simulink model "Copy_2_of_canceshi"  (Simulink 8.8)
settings: Solver=ode4  StartTime=0.0  StopTime=inf  FixedStep=0.1  RelTol=1e-3  EnableMultiTasking=on
undefined symbols (not defined in the file or in its folder): bit, Standard
libraries: slrtlib x21, slrtsoftinglib x11
CloseFcn:
  | rtwprivate ssgencode ModelCloseRequest canceshi
settings Model: xpc_rtwmakecfg_data=_xpccanac2pci_  Creator=Administrator  LastModifiedBy=15751  SimulationMode=external
settings SolverCC: EnableConcurrentExecution=on
settings OptimizationCC: BlockReduction=off  OptimizeBlockIOStorage=off  BufferReuse=off  GlobalBufferReuse=off  ExpressionFolding=off  ExpressionDepthLimit=2147483647  LocalBlockOutputs=off  LifeSpan=auto
settings DebuggingCC: SolverPrmCheckMsg=warning
settings HardwareCC: ProdIntDivRoundTo=Zero  ProdEndianess=LittleEndian  ProdLongLongMode=on  ProdHWDeviceType=Generic->32-bit x86 compatible
settings RTWCC: SystemTargetFile=slrt.tlc  TemplateMakefile=slrt_default_tmf  Description=Simulink Real-Time  RTWCompilerOptimization=on

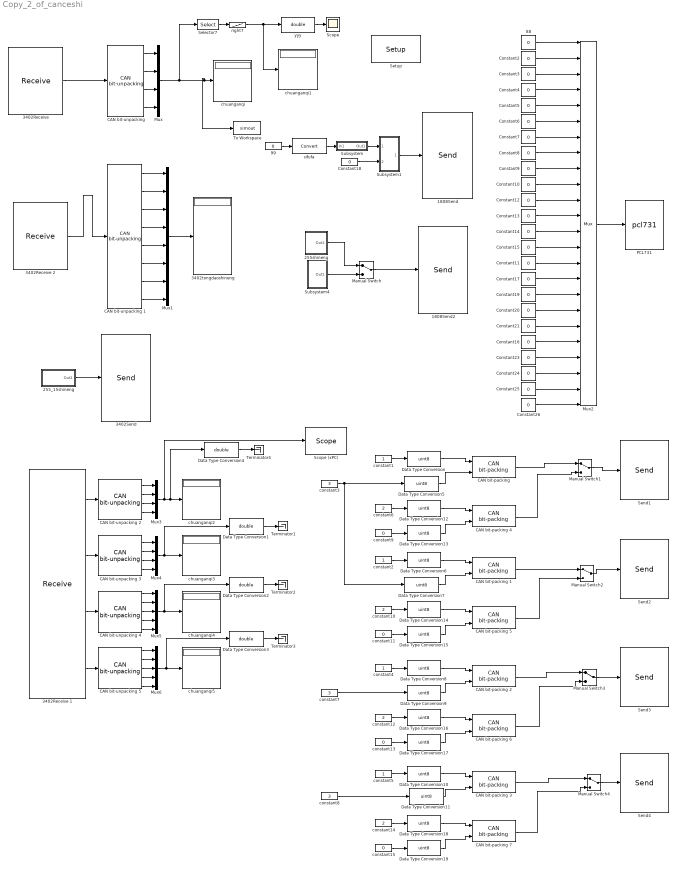
== system Copy_2_of_canceshi ==
  1808Send : slrtsoftinglib/CAN-AC2-PCI SJA 1000/Send   board=1  canPort=CAN 2  range=Standard (11-bit)  ids=[513]  sizes=[8]  output=off  ts=-1  ididx=[4]
  1808Send2 : slrtsoftinglib/CAN-AC2-PCI SJA 1000/Send   board=1  canPort=CAN 2  range=Standard (11-bit)  ids=1537  sizes=[8]  output=off  ts=-1  ididx=[5]
  255_15shineng : Subsystem
  255shineng : Subsystem
  "3402Receive " : slrtsoftinglib/CAN-AC2-PCI SJA 1000/Receive   board=1  canPort=CAN 2  range=Standard (11-bit)  ids=[386]  lengths=0  output=Data  inten=off  ts=-1  ididx=[4]
  3402Receive 1 : slrtsoftinglib/CAN-AC2-PCI SJA 1000/Receive   board=1  canPort=CAN 2  range=Standard (11-bit)  ids=[1 2 3 4]  lengths=8  output=Data  inten=off  ts=-1  ididx=[0,1,2,3]
  3402Receive 2 : slrtsoftinglib/CAN-AC2-PCI SJA 1000/Receive   board=1  canPort=CAN 2  range=Standard (11-bit)  ids=1410  lengths=0  output=Data  inten=off  ts=-1  ididx=[5]
  3402Send : slrtsoftinglib/CAN-AC2-PCI SJA 1000/Send   board=1  canPort=CAN 2  range=Standard (11-bit)  ids=[1538]  sizes=[8]  output=off  ts=-1  ididx=[6]
  3402tongdaoshineng : Display
  88 : Constant  Value=0
  99 : Constant  Value=0
  CAN bit-packing {,1..7} (8 alike) : slrtlib/CAN/Utilities/CAN bit-packing   bitpatterns={ [0:7] [8:15] }
  "CAN bit-unpacking " : slrtlib/CAN/Utilities/CAN bit-unpacking   bitpatterns={ [0:15],[16:31],[32:47],[48:63] }  dtypes={ 'uint16','uint16','uint16','uint16' }
  CAN bit-unpacking 1 : slrtlib/CAN/Utilities/CAN bit-unpacking   bitpatterns={ [0:7],[8:15],[16:23],[24:31],[32:39],[40:47],[48:55],[56:63] }  dtypes={ 'uint8','uint8','uint8','uint8','uint8','uint8','uint8','uint8' }
  CAN bit-unpacking 2 : slrtlib/CAN/Utilities/CAN bit-unpacking   bitpatterns={ [0:7],[8:15],[16:23],[24:31]}  dtypes={ 'uint8','uint8','uint8','uint8' }
  CAN bit-unpacking 3 : slrtlib/CAN/Utilities/CAN bit-unpacking   bitpatterns={ [0:7],[8:15],[16:23],[24:31]}  dtypes={ 'uint8','uint8','uint8','uint8' }
  CAN bit-unpacking 4 : slrtlib/CAN/Utilities/CAN bit-unpacking   bitpatterns={ [0:7],[8:15],[16:23],[24:31],[32:39]}  dtypes={ 'uint8','uint8','uint8','uint8','uint8' }
  CAN bit-unpacking 5 : slrtlib/CAN/Utilities/CAN bit-unpacking   bitpatterns={ [0:7],[8:15],[16:23],[24:31],[32:39]}  dtypes={ 'uint8','uint8','uint8','uint8','uint8' }
  Constant{2..21,23..26} (24 alike) : Constant  Value=0
  Data Type Conversion{,5..19} (16 alike) : DataTypeConversion  OutDataTypeStr=uint8
  Data Type Conversion{1..4} (4 alike) : DataTypeConversion  OutDataTypeStr=double
  Manual Switch{,1..4} (5 alike) : ManualSwitch
  Mux : Mux
  Mux1 : Mux  Inputs=8
  Mux2 : Mux  Inputs=24
  Mux3 : Mux
  Mux4 : Mux
  Mux5 : Mux  Inputs=5
  Mux6 : Mux  Inputs=5
  PCL731 : S-Function  FunctionName=pcl731  Parameters=BaseAddress, [SampleTime SampleOffset]  SFunctionDeploymentMode=off  EnableBusSupport=off  mask(PCL731){sBaseAddr=0x208, Sample=-1}
      mask prompts: sBaseAddr "PCL_731 ADRESS :"; Sample "Sample Time:"
      mask help:
      | PCL-731
      | Advantech
      | Analog Input
      mask init:
      | BaseAddress = 768;SampleTime = 0.001; SampleOffset = 0;
      | sampleLength = length (Sample);
      | %if (sampleLength > 2)
      | %  error ('Sample length vector cannot exceed two elements');
      | %end
      | if (sampleLength == 2)
      |   SampleTime = Sample(1);
      |   SampleOffset = Sample(2);
      | else
      |   SampleTime = Sample(1);
      |   SampleOffset = 0;
      | end
      | 
      | sBaseAddr(find(sBaseAddr=='''')) = [];
      | index = findstr(lower(sBaseAddr),'0x');
      | if ~isempty(index) & index==1
      |   BaseAddr = sBaseAddr(3:end);
      |   baLength = length (BaseAddr);
      |   baseStringMember = [abs('0'):abs('9'),abs('a'):abs('f'),abs('A'):abs('F')];
      |   for i = 1:baLength
      |  %   if ~ismember(BaseAddr(i),baseStringMember)
      |  %     error ('Invalid character in hexadecimal string');
      |  %   end
      |   end
      |   BaseAddress = hex2dec(BaseAddr);
      | else
      |   BaseAddrress = str2num(BaseAddr);
      | end
      mask Display:
      | fprintf('PCL731\n\nSample time:\n%g\nBaseAdress:\n%s', Sample,sBaseAddr)
      | port_label('input',1,'24');
      | port_label('output',1,'24');
  Scope : Scope
  "Scope (xPC) " : slrtlib/Displays and Logging/Scope   scopeno=1  scopetype=Target  autostart=on  viewmode=Numerical  formatstr='%15.6f'  grid=on  ylimits=[0,0]  nosamples=250  noprepostsamples=0  interleave=1  triggermode=FreeRun  triggersignal=1  trigsignalfromport=off  triggerlevel=0.0  triggerslope=Either  triggerscope=1  triggersample=0  filename=data.dat  mode=Lazy  writesize=512  autorestart=off  dynamicfilemode=off  maxwritefilesize=512*1024^2
  Selector7 : Selector  IndexOptions=Index vector (dialog)  Indices=1  OutputSizes=1
  Send1 : slrtsoftinglib/CAN-AC2-PCI SJA 1000/Send   board=1  canPort=CAN 2  range=Standard (11-bit)  ids=1  sizes=[8]  output=off  ts=-1  ididx=[0]
  Send2 : slrtsoftinglib/CAN-AC2-PCI SJA 1000/Send   board=1  canPort=CAN 2  range=Standard (11-bit)  ids=2  sizes=[8]  output=off  ts=-1  ididx=[1]
  Send3 : slrtsoftinglib/CAN-AC2-PCI SJA 1000/Send   board=1  canPort=CAN 2  range=Standard (11-bit)  ids=3  sizes=[8]  output=off  ts=-1  ididx=[2]
  Send4 : slrtsoftinglib/CAN-AC2-PCI SJA 1000/Send   board=1  canPort=CAN 2  range=Standard (11-bit)  ids=4  sizes=[8]  output=off  ts=-1  ididx=[3]
  "Setup " : slrtsoftinglib/CAN-AC2-PCI SJA 1000/Setup   board=1  can1bus=Highspeed (ISO 11898)  can1Baudrate=500 kBaud  can1UserBR=[1,1,4,3]  can2bus=Highspeed (ISO 11898)  can2Baudrate=500 kBaud  can2UserBR=[1,1,4,3]  init=[]  term=[]  bus_off_out=off  bus_off_rec=Off  ioBaseAddress=-1
  Subsystem : Subsystem
  Subsystem1 : Subsystem
  Subsystem4 : Subsystem
  Terminator{1..4} (4 alike) : Terminator
  To Workspace : ToWorkspace  VariableName=simout  SampleTime=-1
  chuanganqi{,1..5} (6 alike) : Display
  constant{1..2,4..5} (4 alike) : Constant
  constant{6,10,12,14} (4 alike) : Constant  Value=2
  constant{9,11,13,15} (4 alike) : Constant  Value=0
  constant3 : Constant  Value=3
  constant7 : Constant  Value=3
  constant8 : Constant  Value=3
  right7 : Lookup  InputValues=[1243 3786]  Table=[0 3200]  LookUpMeth=Interpolation-Use End Values  SaturateOnIntegerOverflow=on
  sifufa : DataTypeConversion
  yyy : DataTypeConversion  OutDataTypeStr=double
  wires:
  255_15shineng/1(Out1) -> 3402Send/1
  Mux2/1 -> PCL731/1
  88/1 -> Mux2/1
  Constant2/1 -> Mux2/2
  Constant3/1 -> Mux2/3
  Constant4/1 -> Mux2/4
  Constant5/1 -> Mux2/5
  Constant6/1 -> Mux2/6
  Constant7/1 -> Mux2/7
  Constant8/1 -> Mux2/8
  Constant9/1 -> Mux2/9
  Constant10/1 -> Mux2/10
  Constant11/1 -> Mux2/15
  Constant15/1 -> Mux2/14
  Constant14/1 -> Mux2/13
  Constant13/1 -> Mux2/12
  Constant12/1 -> Mux2/11
  Constant16/1 -> Mux2/20
  Constant21/1 -> Mux2/19
  Constant20/1 -> Mux2/18
  Constant19/1 -> Mux2/17
  Constant17/1 -> Mux2/16
  Constant26/1 -> Mux2/24
  Constant25/1 -> Mux2/23
  Constant24/1 -> Mux2/22
  Constant23/1 -> Mux2/21
  3402Receive 1/1 -> CAN bit-unpacking 2/1
  3402Receive 1/2 -> CAN bit-unpacking 3/1
  3402Receive 1/3 -> CAN bit-unpacking 4/1
  3402Receive 1/4 -> CAN bit-unpacking 5/1
  CAN bit-unpacking 2/1 -> Mux3/1
  CAN bit-unpacking 2/2 -> Mux3/2
  CAN bit-unpacking 2/3 -> Mux3/3
  CAN bit-unpacking 2/4 -> Mux3/4
  CAN bit-unpacking 3/1 -> Mux4/1
  CAN bit-unpacking 3/2 -> Mux4/2
  CAN bit-unpacking 3/3 -> Mux4/3
  CAN bit-unpacking 3/4 -> Mux4/4
  CAN bit-unpacking 4/1 -> Mux5/1
  CAN bit-unpacking 4/2 -> Mux5/2
  CAN bit-unpacking 4/3 -> Mux5/3
  CAN bit-unpacking 4/4 -> Mux5/4
  CAN bit-unpacking 4/5 -> Mux5/5
  CAN bit-unpacking 5/1 -> Mux6/1
  CAN bit-unpacking 5/2 -> Mux6/2
  CAN bit-unpacking 5/3 -> Mux6/3
  CAN bit-unpacking 5/4 -> Mux6/4
  CAN bit-unpacking 5/5 -> Mux6/5
  Mux3/1 -> chuanganqi2/1, Data Type Conversion4/1, "Scope (xPC) "/1
  Mux4/1 -> chuanganqi3/1, Data Type Conversion1/1
  Mux5/1 -> chuanganqi4/1, Data Type Conversion2/1
  Mux6/1 -> chuanganqi5/1, Data Type Conversion3/1
  Data Type Conversion1/1 -> Terminator1/1
  Data Type Conversion2/1 -> Terminator2/1
  Data Type Conversion3/1 -> Terminator3/1
  Data Type Conversion4/1 -> Terminator4/1
  constant1/1 -> Data Type Conversion/1
  Data Type Conversion/1 -> "CAN bit-packing "/1
  Data Type Conversion5/1 -> "CAN bit-packing "/2
  constant2/1 -> Data Type Conversion6/1
  Data Type Conversion6/1 -> CAN bit-packing 1/1
  Data Type Conversion7/1 -> CAN bit-packing 1/2
  constant4/1 -> Data Type Conversion8/1
  Data Type Conversion8/1 -> CAN bit-packing 2/1
  Data Type Conversion9/1 -> CAN bit-packing 2/2
  constant5/1 -> Data Type Conversion10/1
  Data Type Conversion10/1 -> CAN bit-packing 3/1
  Data Type Conversion11/1 -> CAN bit-packing 3/2
  constant7/1 -> Data Type Conversion9/1
  constant8/1 -> Data Type Conversion11/1
  "3402Receive "/1 -> "CAN bit-unpacking "/1
  "CAN bit-unpacking "/1 -> Mux/1
  "CAN bit-unpacking "/2 -> Mux/2
  "CAN bit-unpacking "/3 -> Mux/3
  "CAN bit-unpacking "/4 -> Mux/4
  CAN bit-unpacking 1/1 -> Mux1/1
  CAN bit-unpacking 1/2 -> Mux1/2
  CAN bit-unpacking 1/3 -> Mux1/3
  CAN bit-unpacking 1/4 -> Mux1/4
  CAN bit-unpacking 1/5 -> Mux1/5
  CAN bit-unpacking 1/6 -> Mux1/6
  CAN bit-unpacking 1/7 -> Mux1/7
  CAN bit-unpacking 1/8 -> Mux1/8
  3402Receive 2/1 -> CAN bit-unpacking 1/1
  Mux/1 -> Selector7/1, chuanganqi/1, To Workspace/1
  Mux1/1 -> 3402tongdaoshineng/1
  Selector7/1 -> right7/1
  yyy/1 -> Scope/1
  Constant18/1 -> Subsystem1/2(In2)
  Subsystem1/1(Out1) -> 1808Send/1
  Subsystem/1(Out1) -> Subsystem1/1(In1)
  99/1 -> sifufa/1
  sifufa/1 -> Subsystem/1(In1)
  Manual Switch/1 -> 1808Send2/1
  255shineng/1(Out1) -> Manual Switch/1
  Subsystem4/1(Out1) -> Manual Switch/2
  right7/1 -> yyy/1, chuanganqi1/1
  constant6/1 -> Data Type Conversion12/1
  Data Type Conversion12/1 -> CAN bit-packing 4/1
  Data Type Conversion13/1 -> CAN bit-packing 4/2
  constant9/1 -> Data Type Conversion13/1
  constant3/1 -> Data Type Conversion5/1, Data Type Conversion7/1
  constant10/1 -> Data Type Conversion14/1
  Data Type Conversion14/1 -> CAN bit-packing 5/1
  Data Type Conversion15/1 -> CAN bit-packing 5/2
  constant11/1 -> Data Type Conversion15/1
  constant12/1 -> Data Type Conversion16/1
  Data Type Conversion16/1 -> CAN bit-packing 6/1
  Data Type Conversion17/1 -> CAN bit-packing 6/2
  constant13/1 -> Data Type Conversion17/1
  constant14/1 -> Data Type Conversion18/1
  Data Type Conversion18/1 -> CAN bit-packing 7/1
  Data Type Conversion19/1 -> CAN bit-packing 7/2
  constant15/1 -> Data Type Conversion19/1
  CAN bit-packing 4/1 -> Manual Switch1/2
  CAN bit-packing 5/1 -> Manual Switch2/2
  CAN bit-packing 6/1 -> Manual Switch3/2
  CAN bit-packing 7/1 -> Manual Switch4/2
  "CAN bit-packing "/1 -> Manual Switch1/1
  Manual Switch1/1 -> Send1/1
  Manual Switch2/1 -> Send2/1
  CAN bit-packing 1/1 -> Manual Switch2/1
  Manual Switch3/1 -> Send3/1
  CAN bit-packing 2/1 -> Manual Switch3/1
  CAN bit-packing 3/1 -> Manual Switch4/1
  Manual Switch4/1 -> Send4/1

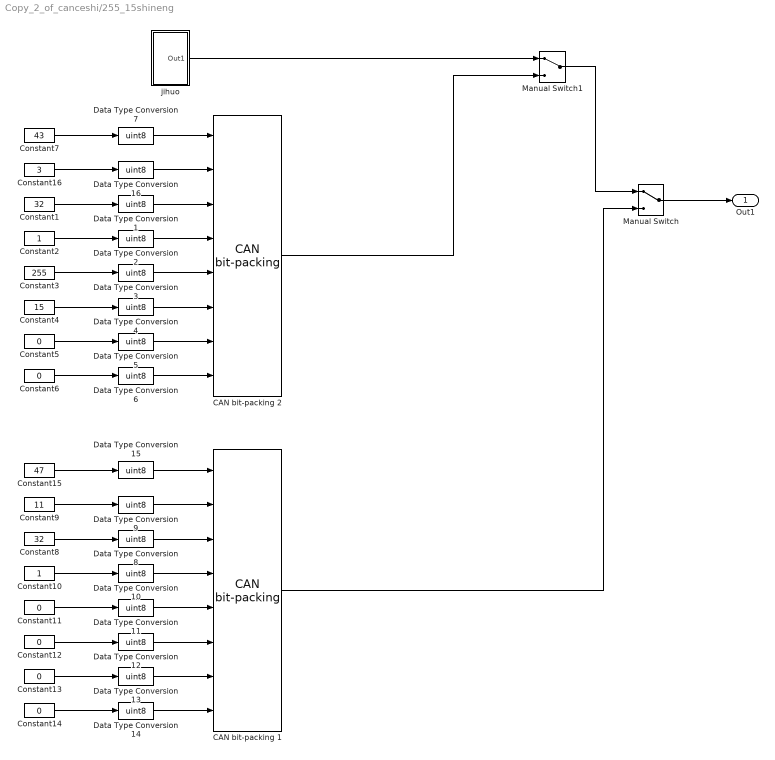
== system Copy_2_of_canceshi/255_15shineng ==
  CAN bit-packing 1 : slrtlib/CAN/Utilities/CAN bit-packing   bitpatterns={ [0:7],[8:15],[16:23],[24:31],[32:39],[40:47],[48:55],[56:63] }
  CAN bit-packing 2 : slrtlib/CAN/Utilities/CAN bit-packing   bitpatterns={ [0:7],[8:15],[16:23],[24:31],[32:39],[40:47],[48:55],[56:63] }
  Constant1 : Constant  Value=32
  Constant10 : Constant
  Constant{5..6,11..14} (6 alike) : Constant  Value=0
  Constant15 : Constant  Value=47
  Constant16 : Constant  Value=3
  Constant2 : Constant
  Constant3 : Constant  Value=255
  Constant4 : Constant  Value=15
  Constant7 : Constant  Value=43
  Constant8 : Constant  Value=32
  Constant9 : Constant  Value=11
  Data Type Conversion{1..16} (16 alike) : DataTypeConversion  OutDataTypeStr=uint8
  Manual Switch : ManualSwitch
  Manual Switch1 : ManualSwitch
  jihuo : Subsystem
  Out1 : Outport
  wires:
  Data Type Conversion7/1 -> CAN bit-packing 2/1
  Data Type Conversion16/1 -> CAN bit-packing 2/2
  Data Type Conversion1/1 -> CAN bit-packing 2/3
  Data Type Conversion2/1 -> CAN bit-packing 2/4
  Data Type Conversion3/1 -> CAN bit-packing 2/5
  Data Type Conversion4/1 -> CAN bit-packing 2/6
  Data Type Conversion5/1 -> CAN bit-packing 2/7
  Data Type Conversion6/1 -> CAN bit-packing 2/8
  Constant7/1 -> Data Type Conversion7/1
  Constant16/1 -> Data Type Conversion16/1
  Constant1/1 -> Data Type Conversion1/1
  Constant2/1 -> Data Type Conversion2/1
  Constant3/1 -> Data Type Conversion3/1
  Constant4/1 -> Data Type Conversion4/1
  Constant5/1 -> Data Type Conversion5/1
  Constant6/1 -> Data Type Conversion6/1
  Data Type Conversion15/1 -> CAN bit-packing 1/1
  Data Type Conversion9/1 -> CAN bit-packing 1/2
  Data Type Conversion8/1 -> CAN bit-packing 1/3
  Data Type Conversion10/1 -> CAN bit-packing 1/4
  Data Type Conversion11/1 -> CAN bit-packing 1/5
  Data Type Conversion12/1 -> CAN bit-packing 1/6
  Data Type Conversion13/1 -> CAN bit-packing 1/7
  Data Type Conversion14/1 -> CAN bit-packing 1/8
  Constant15/1 -> Data Type Conversion15/1
  Constant9/1 -> Data Type Conversion9/1
  Constant8/1 -> Data Type Conversion8/1
  Constant10/1 -> Data Type Conversion10/1
  Constant11/1 -> Data Type Conversion11/1
  Constant12/1 -> Data Type Conversion12/1
  Constant13/1 -> Data Type Conversion13/1
  Constant14/1 -> Data Type Conversion14/1
  CAN bit-packing 1/1 -> Manual Switch/2
  CAN bit-packing 2/1 -> Manual Switch1/2
  Manual Switch/1 -> Out1/1
  jihuo/1(Out1) -> Manual Switch1/1
  Manual Switch1/1 -> Manual Switch/1

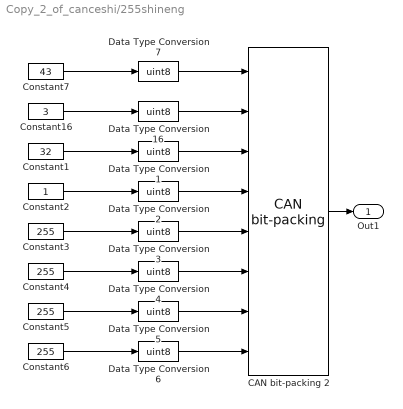
== system Copy_2_of_canceshi/255shineng ==
  CAN bit-packing 2 : slrtlib/CAN/Utilities/CAN bit-packing   bitpatterns={ [0:7],[8:15],[16:23],[24:31],[32:39],[40:47],[48:55],[56:63] }
  Constant1 : Constant  Value=32
  Constant16 : Constant  Value=3
  Constant2 : Constant
  Constant{3..6} (4 alike) : Constant  Value=255
  Constant7 : Constant  Value=43
  Data Type Conversion{1..7,16} (8 alike) : DataTypeConversion  OutDataTypeStr=uint8
  Out1 : Outport
  wires:
  CAN bit-packing 2/1 -> Out1/1
  Constant6/1 -> Data Type Conversion6/1
  Constant5/1 -> Data Type Conversion5/1
  Constant4/1 -> Data Type Conversion4/1
  Constant3/1 -> Data Type Conversion3/1
  Constant2/1 -> Data Type Conversion2/1
  Constant1/1 -> Data Type Conversion1/1
  Constant16/1 -> Data Type Conversion16/1
  Constant7/1 -> Data Type Conversion7/1
  Data Type Conversion6/1 -> CAN bit-packing 2/8
  Data Type Conversion5/1 -> CAN bit-packing 2/7
  Data Type Conversion4/1 -> CAN bit-packing 2/6
  Data Type Conversion3/1 -> CAN bit-packing 2/5
  Data Type Conversion2/1 -> CAN bit-packing 2/4
  Data Type Conversion1/1 -> CAN bit-packing 2/3
  Data Type Conversion16/1 -> CAN bit-packing 2/2
  Data Type Conversion7/1 -> CAN bit-packing 2/1

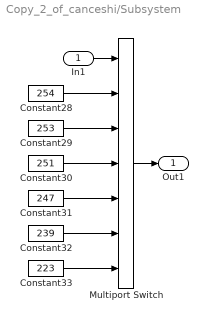
== system Copy_2_of_canceshi/Subsystem ==
  In1 : Inport
  Constant28 : Constant  Value=254
  Constant29 : Constant  Value=253
  Constant30 : Constant  Value=251
  Constant31 : Constant  Value=247
  Constant32 : Constant  Value=239
  Constant33 : Constant  Value=223
  Multiport Switch : MultiPortSwitch  Inputs=6
  Out1 : Outport
  wires:
  Constant28/1 -> Multiport Switch/2
  Constant29/1 -> Multiport Switch/3
  Constant30/1 -> Multiport Switch/4
  Constant31/1 -> Multiport Switch/5
  Constant32/1 -> Multiport Switch/6
  Constant33/1 -> Multiport Switch/7
  In1/1 -> Multiport Switch/1
  Multiport Switch/1 -> Out1/1

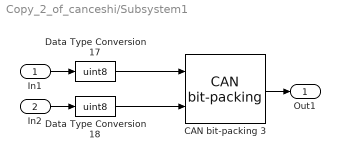
== system Copy_2_of_canceshi/Subsystem1 ==
  In1 : Inport
  In2 : Inport  Port=2
  CAN bit-packing 3 : slrtlib/CAN/Utilities/CAN bit-packing   bitpatterns={ [0:7],[8:15] }
  Data Type Conversion17 : DataTypeConversion  OutDataTypeStr=uint8
  Data Type Conversion18 : DataTypeConversion  OutDataTypeStr=uint8
  Out1 : Outport
  wires:
  Data Type Conversion17/1 -> CAN bit-packing 3/1
  Data Type Conversion18/1 -> CAN bit-packing 3/2
  In1/1 -> Data Type Conversion17/1
  CAN bit-packing 3/1 -> Out1/1
  In2/1 -> Data Type Conversion18/1

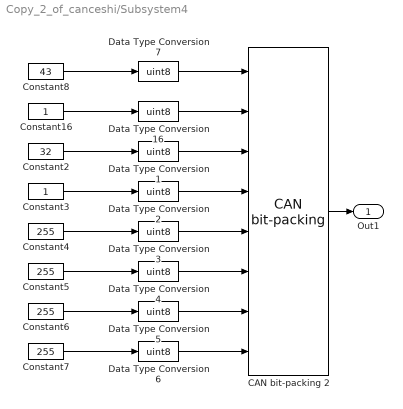
== system Copy_2_of_canceshi/Subsystem4 ==
  CAN bit-packing 2 : slrtlib/CAN/Utilities/CAN bit-packing   bitpatterns={ [0:7],[8:15],[16:23],[24:31],[32:39],[40:47],[48:55],[56:63] }
  Constant16 : Constant
  Constant2 : Constant  Value=32
  Constant3 : Constant
  Constant{4..7} (4 alike) : Constant  Value=255
  Constant8 : Constant  Value=43
  Data Type Conversion{1..7,16} (8 alike) : DataTypeConversion  OutDataTypeStr=uint8
  Out1 : Outport
  wires:
  Data Type Conversion7/1 -> CAN bit-packing 2/1
  Data Type Conversion16/1 -> CAN bit-packing 2/2
  Data Type Conversion1/1 -> CAN bit-packing 2/3
  Data Type Conversion2/1 -> CAN bit-packing 2/4
  Data Type Conversion3/1 -> CAN bit-packing 2/5
  Data Type Conversion4/1 -> CAN bit-packing 2/6
  Data Type Conversion5/1 -> CAN bit-packing 2/7
  Data Type Conversion6/1 -> CAN bit-packing 2/8
  Constant8/1 -> Data Type Conversion7/1
  Constant16/1 -> Data Type Conversion16/1
  Constant2/1 -> Data Type Conversion1/1
  Constant3/1 -> Data Type Conversion2/1
  Constant4/1 -> Data Type Conversion3/1
  Constant5/1 -> Data Type Conversion4/1
  Constant6/1 -> Data Type Conversion5/1
  Constant7/1 -> Data Type Conversion6/1
  CAN bit-packing 2/1 -> Out1/1

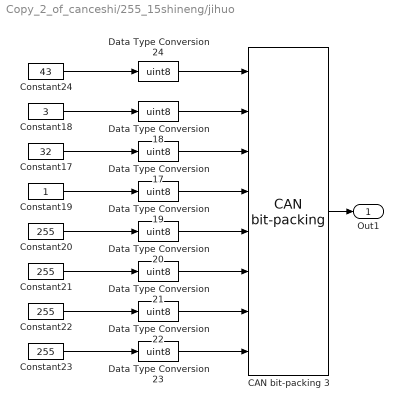
== system Copy_2_of_canceshi/255_15shineng/jihuo ==
  CAN bit-packing 3 : slrtlib/CAN/Utilities/CAN bit-packing   bitpatterns={ [0:7],[8:15],[16:23],[24:31],[32:39],[40:47],[48:55],[56:63] }
  Constant17 : Constant  Value=32
  Constant18 : Constant  Value=3
  Constant19 : Constant
  Constant{20..23} (4 alike) : Constant  Value=255
  Constant24 : Constant  Value=43
  Data Type Conversion{17..24} (8 alike) : DataTypeConversion  OutDataTypeStr=uint8
  Out1 : Outport
  wires:
  Data Type Conversion24/1 -> CAN bit-packing 3/1
  Data Type Conversion18/1 -> CAN bit-packing 3/2
  Data Type Conversion17/1 -> CAN bit-packing 3/3
  Data Type Conversion19/1 -> CAN bit-packing 3/4
  Data Type Conversion20/1 -> CAN bit-packing 3/5
  Data Type Conversion21/1 -> CAN bit-packing 3/6
  Data Type Conversion22/1 -> CAN bit-packing 3/7
  Data Type Conversion23/1 -> CAN bit-packing 3/8
  Constant24/1 -> Data Type Conversion24/1
  Constant18/1 -> Data Type Conversion18/1
  Constant17/1 -> Data Type Conversion17/1
  Constant19/1 -> Data Type Conversion19/1
  Constant20/1 -> Data Type Conversion20/1
  Constant21/1 -> Data Type Conversion21/1
  Constant22/1 -> Data Type Conversion22/1
  Constant23/1 -> Data Type Conversion23/1
  CAN bit-packing 3/1 -> Out1/1
